simulink model "Experiment_AERO_pitch_channel"  (Simulink 9.1)
settings: Solver=ode4  StartTime=0.0  StopTime=35  FixedStep=0.001  RelTol=1e-3  EnableMultiTasking=on
InitFcn:
  | Parameters_and_initial_conditions
values from neighbouring files (symbols this model uses):
  a1 = -Ksp/Jp    (= -3.27334590734)    [Parameters_and_initial_conditions.m]
  a2 = -Dp/Jp    (= -0.354944459971)    [Parameters_and_initial_conditions.m]
  alpha1 = 0.5    [Parameters_and_initial_conditions.m]
  alpha2 = 0.25    [Parameters_and_initial_conditions.m]
  beta1 = 1    [Parameters_and_initial_conditions.m]
  beta1_HGOB = 3/eps    (= 300)    [Parameters_and_initial_conditions.m]
  beta2 = 1/(2*stepsize^0.5)    (= 1.58113883008)    [Parameters_and_initial_conditions.m]
  beta2_HGOB = 3/(eps^2)    (= 30000)    [Parameters_and_initial_conditions.m]
  beta3 = 2/(25*stepsize^1.2)    (= 1.26791455397)    [Parameters_and_initial_conditions.m]
  beta3_HGOB = 1/(eps^3)    (= 1000000)    [Parameters_and_initial_conditions.m]
  delta = 10    [Parameters_and_initial_conditions.m]
  Dp = 0.007768621416960    (= 0.00776862141696)    [Parameters_and_initial_conditions.m]
  Dp_static = Dp*0.05    (= 0.000388431070848)    [Parameters_and_initial_conditions.m]
  Dy = 0.0220    (= 0.022)    [Parameters_and_initial_conditions.m]
  Jp = J_body + 2*J_prop    (= 0.0218868648283)    [Parameters_and_initial_conditions.m]
  Jy = J_body + 2*J_prop + J_yoke    (= 0.0219920648283)    [Parameters_and_initial_conditions.m]
  kd = 3    [Parameters_and_initial_conditions.m]
  kp = 5    [Parameters_and_initial_conditions.m]
  Kpp = 9.971955650940002e-04    (= 0.000997195565094)    [Parameters_and_initial_conditions.m]
  Kpy = 0.0021    [Parameters_and_initial_conditions.m]
  Ksp = 0.071643279410402    (= 0.0716432794104)    [Parameters_and_initial_conditions.m]
  Kyp = -0.0027    [Parameters_and_initial_conditions.m]
  Kyy = 0.0022    [Parameters_and_initial_conditions.m]
  PitchAxisEnable = 1    [Parameters_and_initial_conditions.m]
  PitchMotorEnable = 1    [Parameters_and_initial_conditions.m]
  psi_dot_initial = 0.0    (= 0)    [Parameters_and_initial_conditions.m]
  psi_initial = 0.0    (= 0)    [Parameters_and_initial_conditions.m]
  theta_dot_initial = 0.0    (= 0)    [Parameters_and_initial_conditions.m]
  theta_initial = 0.0    (= 0)    [Parameters_and_initial_conditions.m]
  YawAxisEnable = 0    [Parameters_and_initial_conditions.m]
  YawMotorEnable = 0    [Parameters_and_initial_conditions.m]
libraries: quarc_library x9, simulink_extras x5, quanser_aero x1
settings Model: Creator=MLevis  LastModifiedBy=DELL  SimulationMode=external  ExtModeTrigDuration=5000
settings SolverCC: PositivePriorityOrder=on
settings DataIOCC: LimitDataPoints=on
settings DebuggingCC: UnderspecifiedInitializationDetection=Simplified  MergeDetectMultiDrivingBlocksExec=error  SolverPrmCheckMsg=warning
settings RTWCC: SystemTargetFile=quarc_win64.tlc  TemplateMakefile=quarc_default_tmf  Description=QUARC Win64 Target
settings STFCustomTargetCC: TargetPreCompLibLocation=C:\PROGRA~3\QUARC\lib\2018a\win64\release  ConcurrentExecutionCompliant=on  GeneratePreprocessorConditionals=Disable all  SystemTargetFile=quarc_win64.tlc
settings GRTTargetCC: TargetPreCompLibLocation=C:\PROGRA~3\QUARC\lib\2018a\win64\release  ParMdlRefBuildCompliant=off  CompOptLevelCompliant=off  GeneratePreprocessorConditionals=Disable all  MatFileLogging=off  CPPClassGenCompliant=off  UseToolchainInfoCompliant=off  ExtMode=on  ExtModeMexFile=quarc_comm
settings ConfigComp: CovSFcnEnable=off

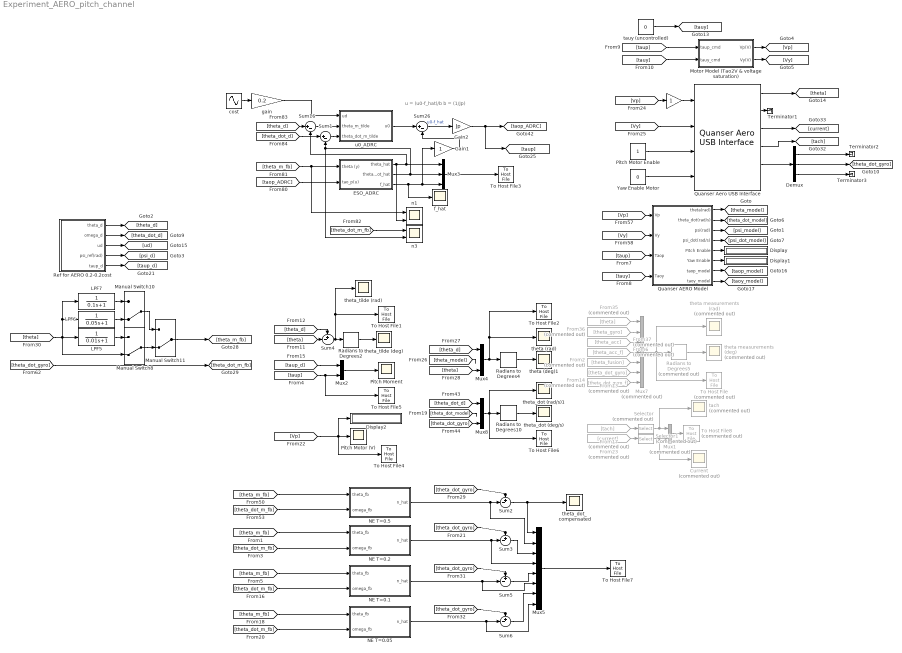
== system Experiment_AERO_pitch_channel ==
  note: u = (u0-f_hat)/b
      | b = (1/Jp)
  " " : Gain
  Current : Scope  Commented=on
  Demux : Demux  Outputs=3
  Display : Display
  Display1 : Display
  Display2 : Display
  ESO_ADRC : Subsystem
  From13 : From  Commented=on  GotoTag=theta_dot_gyro
  From14 : From  Commented=on  GotoTag=theta_dot_gyro_f
  From17 : From  Commented=on  GotoTag=tach
  From2 : From  Commented=on  GotoTag=theta_fusion
  From23 : From  Commented=on  GotoTag=current
  From35 : From  Commented=on  GotoTag=theta
  From36 : From  Commented=on  GotoTag=theta_gyro
  From37 : From  Commented=on  GotoTag=theta_acc
  From6 : From  Commented=on  GotoTag=theta_acc_f
  Gain1 : Gain
  Gain2 : Gain  Gain=Jp
  LPF5 : TransferFcn  Denominator=[0.01 1]
  LPF6 : TransferFcn  Denominator=[0.05 1]
  LPF7 : TransferFcn  Denominator=[0.1 1]
  Manual Switch10 : ManualSwitch  CurrentSetting=0
  Manual Switch11 : ManualSwitch  CurrentSetting=0
  Manual Switch8 : ManualSwitch  CurrentSetting=0
  Motor Model (Tao2V & voltage saturation) : Subsystem
  Mux1 : Mux  Commented=on  Inputs=2
  Mux2 : Mux  Inputs=2
  Mux3 : Mux  Inputs=3
  Mux4 : Mux  Inputs=3
  Mux5 : Mux  Inputs=8
  Mux7 : Mux  Commented=on  Inputs=7
  Mux8 : Mux  Inputs=3
  NE T=0.05 : Subsystem
  NE T=0.1 : Subsystem
  NE T=0.2 : Subsystem
  NE T=0.5 : Subsystem
  Pitch Moment : Scope
  Pitch Motor (V) : Scope
  Pitch Motor Enable : Constant
  Quanser AERO Model : Subsystem
  Quanser Aero USB Interface : quanser_aero/Quanser Aero USB Interface
  Radians to Degrees10 : simulink_extras/Transformations/Radians to Degrees
  Radians to Degrees2 : simulink_extras/Transformations/Radians to Degrees
  Radians to Degrees4 : simulink_extras/Transformations/Radians to Degrees
  Radians to Degrees5 : simulink_extras/Transformations/Radians to Degrees  Commented=on
  Ref for AERO 0.2-0.2cost : Subsystem
  Selector : Selector  Commented=on  InputPortWidth=2  IndexOptions=Index vector (dialog)  Indices=[1]  OutputSizes=1
  Selector1 : Selector  Commented=on  InputPortWidth=2  IndexOptions=Index vector (dialog)  Indices=[1]  OutputSizes=1
  Sum1 : Sum  Inputs=|+-
  Sum16 : Sum  Inputs=|+-
  Sum{2..6} (5 alike) : Sum  Inputs=+-|
  Sum26 : Sum  Inputs=|+-
  Terminator1 : Terminator
  Terminator2 : Terminator
  Terminator3 : Terminator
  To Host File : quarc_library/Sinks/To Host/To Host File  Commented=on  file_name=Log_Sensor_Measurements.mat  variable_name=Log_Sensor_Measurements  decimation=1  sample_time=-1  file_format=MAT-file v.5  options=No header or footer  append=off  final_file_name=Log_Sensor_Measurements.mat  bitrate=2000000
  To Host File1 : quarc_library/Sinks/To Host/To Host File  file_name=Log_Tracking_Err.mat  variable_name=Log_Tracking_Err  decimation=1  sample_time=-1  file_format=MAT-file v.5  options=No header or footer  append=off  final_file_name=Log_Tracking_Err.mat  bitrate=2000000
  To Host File2 : quarc_library/Sinks/To Host/To Host File  file_name=Log_Theta_Response.mat  variable_name=Log_Theta_Response  decimation=1  sample_time=-1  file_format=MAT-file v.5  options=No header or footer  append=off  final_file_name=Log_Theta_Response.mat  bitrate=2000000
  To Host File3 : quarc_library/Sinks/To Host/To Host File  file_name=Log_ESO.mat  variable_name=Log_ESO  decimation=1  sample_time=-1  file_format=MAT-file v.5  options=No header or footer  append=off  final_file_name=Log_ESO.mat  bitrate=2000000
  To Host File4 : quarc_library/Sinks/To Host/To Host File  file_name=Log_Input_Voltage.mat  variable_name=Log_Input_Voltage  decimation=1  sample_time=-1  file_format=MAT-file v.5  options=No header or footer  append=off  final_file_name=Log_Input_Voltage.mat  bitrate=2000000
  To Host File5 : quarc_library/Sinks/To Host/To Host File  file_name=Log_Input_Torque.mat  variable_name=Log_Input_Torque  decimation=1  sample_time=-1  file_format=MAT-file v.5  options=No header or footer  append=off  final_file_name=Log_Input_Torque.mat  bitrate=2000000
  To Host File6 : quarc_library/Sinks/To Host/To Host File  file_name=Log_Theta_dot_Response.mat  variable_name=Log_Theta_dot_Response  decimation=1  sample_time=-1  file_format=MAT-file v.5  options=No header or footer  append=off  final_file_name=Log_Theta_dot_Response.mat  bitrate=2000000
  To Host File7 : quarc_library/Sinks/To Host/To Host File  file_name=Log_Theta_dot_NE_estimation.mat  variable_name=Log_Theta_dot_NE_estimation  decimation=1  sample_time=-1  file_format=MAT-file v.5  options=No header or footer  append=off  final_file_name=Log_Theta_dot_NE_estimation.mat  bitrate=2000000
  To Host File8 : quarc_library/Sinks/To Host/To Host File  Commented=on  file_name=Log_Tach_Current.mat  variable_name=Log_Tach_Current  decimation=1  sample_time=-1  file_format=MAT-file v.5  options=No header or footer  append=off  final_file_name=Log_Tach_Current.mat  bitrate=2000000
  Yaw Enable Motor : Constant  Value=0
  cost : Sin  Phase=pi/2  SampleTime=0
  f_hat : Scope
  gain : Gain  Gain=0.2
  n1 : Scope  NumInputPorts=2
  n3 : Scope  NumInputPorts=2
  tach : Scope  Commented=on
  tauy (uncontrolled) : Constant  Value=0
  theta (deg)1 : Scope
  theta (rad) : Scope
  theta measurements (deg) : Scope  Commented=on
  theta measurements (rad) : Scope  Commented=on
  theta_dot (deg/s) : Scope
  theta_dot (rad/s)1 : Scope
  theta_dot_compensated : Scope
  theta_tilde (deg) : Scope
  theta_tilde (rad) : Scope
  u0_ADRC : Subsystem
  wires:
  Quanser AERO Model/3(psi(rad)) -> [psi_model]
  Quanser AERO Model/1(theta(rad)) -> [theta_model]
  Mux2/1 -> Pitch Moment/1
  Quanser AERO Model/2(theta_dot(rad/s)) -> [theta_dot_model]
  Quanser AERO Model/4(psi_dot(rad/s)) -> [psi_dot_model]
  Quanser AERO Model/5(Pitch Enable) -> Display/1
  Quanser AERO Model/6(Yaw Enable) -> Display1/1
  Motor Model (Tao2V & voltage saturation)/1(Vp(V)) -> [Vp]
  Motor Model (Tao2V & voltage saturation)/2(Vy(V)) -> [Vy]
  [tauy] -> Motor Model (Tao2V & voltage saturation)/2(tauy_cmd)
  [taup] -> Motor Model (Tao2V & voltage saturation)/1(taup_cmd)
  [theta_d] -> Sum4/1
  [theta] -> Sum4/2
  Sum4/1 -> To Host File1/1, theta_tilde (rad)/1, Radians to Degrees2/1
  Radians to Degrees2/1 -> theta_tilde (deg)/1
  [taup] -> To Host File5/1, Mux2/2
  [taup_d] -> Mux2/1
  tauy (uncontrolled)/1 -> [tauy]
  [Vp] -> Display2/1, To Host File4/1, Pitch Motor (V)/1
  Quanser Aero USB Interface/5 -> Demux/1
  Yaw Enable Motor/1 -> Quanser Aero USB Interface/4
  Quanser Aero USB Interface/4 -> [tach]
  Quanser Aero USB Interface/1 -> [theta]
  Demux/3 -> Terminator3/1
  Pitch Motor Enable/1 -> Quanser Aero USB Interface/3
  Quanser Aero USB Interface/3 -> [current]
  [Vy] -> Quanser Aero USB Interface/2
  Demux/1 -> Terminator2/1
  Demux/2 -> [theta_dot_gyro]
  Quanser Aero USB Interface/2 -> Terminator1/1
  " "/1 -> Quanser Aero USB Interface/1
  Radians to Degrees4/1 -> theta (deg)1/1
  [theta_model] -> ?
  [theta_d] -> Mux4/1
  [theta] -> Mux4/3
  Quanser AERO Model/7(taop_model) -> [taop_model]
  Quanser AERO Model/8(taoy_model) -> [taoy_model]
  From35/1 -> Mux7/1
  From36/1 -> Mux7/2
  From37/1 -> Mux7/3
  Radians to Degrees5/1 -> theta measurements (deg)/1
  Radians to Degrees10/1 -> theta_dot (deg/s)/1
  [theta_dot_model] -> ?
  Mux8/1 -> Radians to Degrees10/1, To Host File6/1, theta_dot (rad/s)1/1
  [theta_dot_gyro] -> Mux8/3
  [theta_dot_d] -> Mux8/1
  From6/1 -> Mux7/4
  Mux7/1 -> To Host File/1, theta measurements (rad)/1, Radians to Degrees5/1
  [taup] -> Quanser AERO Model/3(Taop)
  [tauy] -> Quanser AERO Model/4(Taoy)
  [Vp] -> Quanser AERO Model/1(Vp)
  [Vy] -> Quanser AERO Model/2(Vy)
  [theta_dot_gyro] -> [theta_dot_m_fb]
  Mux4/1 -> Radians to Degrees4/1, To Host File2/1, theta (rad)/1
  From2/1 -> Mux7/5
  From13/1 -> Mux7/6
  From14/1 -> Mux7/7
  From17/1 -> Selector/1
  Mux1/1 -> To Host File8/1
  From23/1 -> Selector1/1
  Selector/1 -> tach/1, Mux1/1
  Selector1/1 -> Current/1, Mux1/2
  Ref for AERO 0.2-0.2cost/1(theta_d) -> [theta_d]
  Ref for AERO 0.2-0.2cost/2(omega_d) -> [theta_dot_d]
  Ref for AERO 0.2-0.2cost/4(psi_ref(rad)) -> [psi_d]
  Ref for AERO 0.2-0.2cost/3(ud) -> [ud]
  Manual Switch11/1 -> [theta_m_fb]
  [theta] -> LPF5/1, Manual Switch8/2, LPF7/1, LPF6/1
  Ref for AERO 0.2-0.2cost/5(taup_d) -> [taup_d]
  LPF5/1 -> Manual Switch8/1
  LPF6/1 -> Manual Switch10/2
  LPF7/1 -> Manual Switch10/1
  Manual Switch10/1 -> Manual Switch11/1
  Manual Switch8/1 -> Manual Switch11/2
  [Vp] -> " "/1
  ESO_ADRC/3(f_hat) -> f_hat/1, Gain1/1, Mux3/3
  ESO_ADRC/1(theta_hat) -> n1/2, Sum16/2, Mux3/1
  [theta_dot_m_fb] -> n3/1
  u0_ADRC/1(u0) -> Sum26/1
  Gain1/1 -> Sum26/2
  Sum26/1 -> Gain2/1  "u0-f_hat"
  [taop_ADRC] -> ESO_ADRC/2(tao_p(u))
  [theta_d] -> Sum16/1
  ESO_ADRC/2(theta_dot_hat) -> Mux3/2, n3/2, Sum1/2
  Gain2/1 -> [taup], [taop_ADRC]
  [theta_m_fb] -> n1/1, ESO_ADRC/1(theta (y))
  [theta_dot_d] -> Sum1/1
  Sum16/1 -> u0_ADRC/2(theta_m_tilde)
  Sum1/1 -> u0_ADRC/3(theta_dot_m_tilde)
  Mux3/1 -> To Host File3/1
  cost/1 -> gain/1
  gain/1 -> u0_ADRC/1(ud)
  [theta_m_fb] -> NE T=0.5/1(theta_fb)
  [theta_dot_m_fb] -> NE T=0.5/2(omega_fb)
  Sum2/1 -> Mux5/1, theta_dot_compensated/1
  [theta_dot_gyro] -> Sum2/1
  Mux5/1 -> To Host File7/1
  NE T=0.5/1(n_hat) -> Mux5/2, Sum2/2
  [theta_dot_m_fb] -> NE T=0.2/2(omega_fb)
  [theta_m_fb] -> NE T=0.2/1(theta_fb)
  [theta_dot_m_fb] -> NE T=0.1/2(omega_fb)
  [theta_m_fb] -> NE T=0.1/1(theta_fb)
  [theta_dot_m_fb] -> NE T=0.05/2(omega_fb)
  [theta_m_fb] -> NE T=0.05/1(theta_fb)
  [theta_dot_gyro] -> Sum3/1
  [theta_dot_gyro] -> Sum5/1
  NE T=0.2/1(n_hat) -> Mux5/4, Sum3/2
  NE T=0.05/1(n_hat) -> Mux5/8, Sum6/2
  [theta_dot_gyro] -> Sum6/1
  NE T=0.1/1(n_hat) -> Mux5/6, Sum5/2
  Sum3/1 -> Mux5/3
  Sum5/1 -> Mux5/5
  Sum6/1 -> Mux5/7

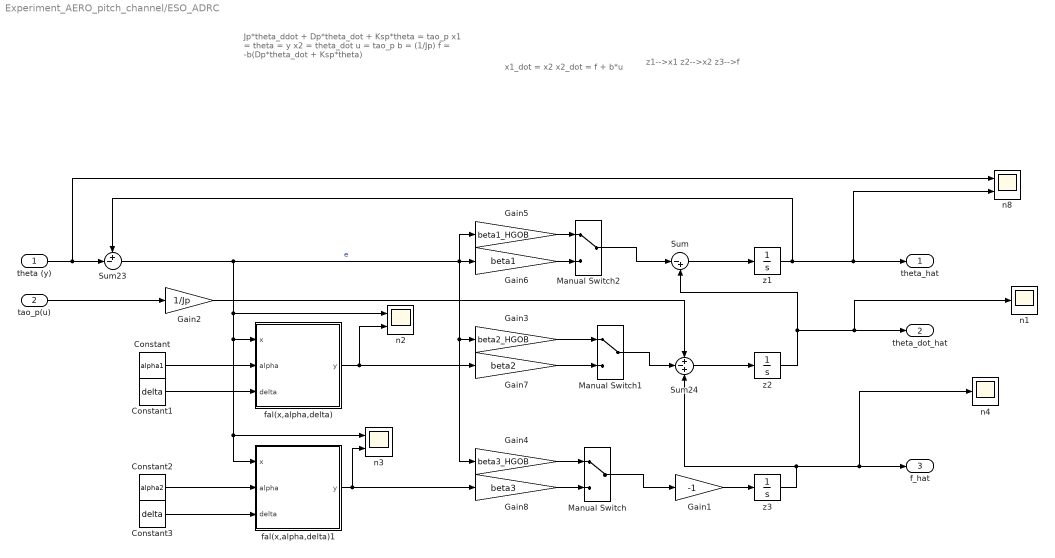
== system Experiment_AERO_pitch_channel/ESO_ADRC ==
  note: z1-->x1
      | z2-->x2
      | z3-->f
  note: x1_dot = x2
      | x2_dot = f + b*u
  note: Jp*theta_ddot + Dp*theta_dot + Ksp*theta = tao_p
      | x1 = theta = y
      | x2 = theta_dot
      | u = tao_p
      | b = (1/Jp)
      | f = -b(Dp*theta_dot + Ksp*theta)
  theta (y) : Inport
  tao_p(u) : Inport  Port=2
  Constant : Constant  Value=alpha1
  Constant1 : Constant  Value=delta
  Constant2 : Constant  Value=alpha2
  Constant3 : Constant  Value=delta
  Gain1 : Gain  Gain=-1
  Gain2 : Gain  Gain=1/Jp
  Gain3 : Gain  Gain=beta2_HGOB
  Gain4 : Gain  Gain=beta3_HGOB
  Gain5 : Gain  Gain=beta1_HGOB
  Gain6 : Gain  Gain=beta1
  Gain7 : Gain  Gain=beta2
  Gain8 : Gain  Gain=beta3
  Manual Switch : ManualSwitch
  Manual Switch1 : ManualSwitch
  Manual Switch2 : ManualSwitch
  Sum : Sum  Inputs=|-+
  Sum23 : Sum  Inputs=+-|
  Sum24 : Sum  Inputs=+-+
  fal(x,alpha,delta) : MATLAB Function  TreatAsAtomicUnit=on
  fal(x,alpha,delta)1 : MATLAB Function  TreatAsAtomicUnit=on
  n1 : Scope
  n2 : Scope  NumInputPorts=2
  n3 : Scope  NumInputPorts=2
  n4 : Scope
  n8 : Scope  NumInputPorts=2
  z1 : Integrator
  z2 : Integrator
  z3 : Integrator
  theta_hat : Outport
  theta_dot_hat : Outport  Port=2
  f_hat : Outport  Port=3
  wires:
  z2/1 -> Sum/2, n1/1, theta_dot_hat/1
  Sum23/1 -> Gain6/1, Gain5/1, Gain3/1, Gain4/1, n2/1, n3/1, fal(x,alpha,delta)1/1(x), fal(x,alpha,delta)/1(x)  "e"
  Gain7/1 -> Manual Switch1/2
  Gain6/1 -> Manual Switch2/2
  z3/1 -> Sum24/3, n4/1, f_hat/1
  Sum24/1 -> z2/1
  Sum/1 -> z1/1
  z1/1 -> n8/2, theta_hat/1, Sum23/1
  Gain8/1 -> Manual Switch/2
  theta (y)/1 -> n8/1, Sum23/2
  tao_p(u)/1 -> Gain2/1
  Gain1/1 -> z3/1
  Gain2/1 -> Sum24/1
  fal(x,alpha,delta)/1(y) -> Gain7/1, n2/2
  Constant/1 -> fal(x,alpha,delta)/2(alpha)
  Constant1/1 -> fal(x,alpha,delta)/3(delta)
  Constant3/1 -> fal(x,alpha,delta)1/3(delta)
  Constant2/1 -> fal(x,alpha,delta)1/2(alpha)
  fal(x,alpha,delta)1/1(y) -> Gain8/1, n3/2
  Gain4/1 -> Manual Switch/1
  Manual Switch/1 -> Gain1/1
  Gain3/1 -> Manual Switch1/1
  Manual Switch1/1 -> Sum24/2
  Gain5/1 -> Manual Switch2/1
  Manual Switch2/1 -> Sum/1

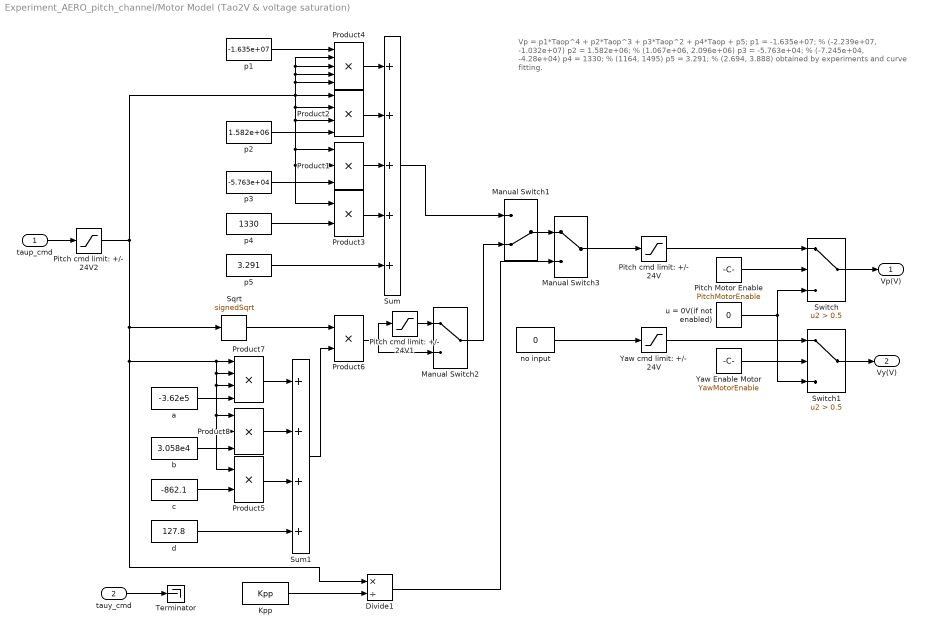
== system Experiment_AERO_pitch_channel/Motor Model (Tao2V & voltage saturation) ==
  note: Vp = p1*Taop^4 + p2*Taop^3 + p3*Taop^2 + p4*Taop + p5;
      | p1 = -1.635e+07; % (-2.239e+07, -1.032e+07)
      | p2 = 1.582e+06; % (1.067e+06, 2.096e+06)
      | p3 = -5.763e+04; % (-7.245e+04, -4.28e+04)
      | p4 = 1330; % (1164, 1495)
      | p5 = 3.291; % (2.694, 3.888)
      |
      | obtained by experiments and curve fitting.
  taup_cmd : Inport
  tauy_cmd : Inport  Port=2
  Divide1 : Product  Inputs=*/
  Kpp : Constant  Value=Kpp
  Manual Switch1 : ManualSwitch  CurrentSetting=0
  Manual Switch2 : ManualSwitch
  Manual Switch3 : ManualSwitch
  Pitch Motor Enable : Constant  Value=PitchMotorEnable
  Pitch cmd limit: +/- 24V : Saturate  UpperLimit=24  LowerLimit=-24
  Pitch cmd limit: +/- 24V1 : Saturate  UpperLimit=24  LowerLimit=0
  Pitch cmd limit: +/- 24V2 : Saturate  UpperLimit=0.05  LowerLimit=0
  Product1 : Product  Inputs=3
  Product2 : Product  Inputs=4
  Product3 : Product
  Product4 : Product  Inputs=5
  Product5 : Product
  Product6 : Product
  Product7 : Product  Inputs=4
  Product8 : Product  Inputs=3
  Sqrt : Sqrt  Operator=signedSqrt  SaturateOnIntegerOverflow=on
  Sum : Sum  Inputs=+++++
  Sum1 : Sum  Inputs=++++
  Switch : Switch  Criteria=u2 > Threshold  Threshold=0.5
  Switch1 : Switch  Criteria=u2 > Threshold  Threshold=0.5
  Terminator : Terminator
  Yaw Enable Motor : Constant  Value=YawMotorEnable
  Yaw cmd limit: +/- 24V : Saturate  UpperLimit=24  LowerLimit=-24
  a : Constant  Value=-3.62e5
  b : Constant  Value=3.058e4
  c : Constant  Value=-862.1
  d : Constant  Value=127.8
  no input : Constant  Value=0
  p1 : Constant  Value=-1.635e+07
  p2 : Constant  Value=1.582e+06
  p3 : Constant  Value=-5.763e+04
  p4 : Constant  Value=1330
  p5 : Constant  Value=3.291
  u = 0V(if not enabled) : Constant  Value=0
  Vp(V) : Outport
  Vy(V) : Outport  Port=2
  wires:
  Pitch Motor Enable/1 -> Switch/2
  Yaw Enable Motor/1 -> Switch1/2
  Switch/1 -> Vp(V)/1
  Switch1/1 -> Vy(V)/1
  Yaw cmd limit: +/- 24V/1 -> Switch1/1
  Pitch cmd limit: +/- 24V/1 -> Switch/1
  u = 0V(if not enabled)/1 -> Switch1/3, Switch/3
  tauy_cmd/1 -> Terminator/1
  p2/1 -> Product2/4
  no input/1 -> Yaw cmd limit: +/- 24V/1
  Product2/1 -> Sum/2
  p3/1 -> Product1/3
  p4/1 -> Product3/2
  Kpp/1 -> Divide1/2
  Product1/1 -> Sum/3
  Product3/1 -> Sum/4
  p5/1 -> Sum/5
  Sum/1 -> Manual Switch1/1
  Product4/1 -> Sum/1
  p1/1 -> Product4/1
  Manual Switch3/1 -> Pitch cmd limit: +/- 24V/1
  a/1 -> Product7/4
  b/1 -> Product8/3
  Sum1/1 -> Product6/2
  Sqrt/1 -> Product6/1
  Product6/1 -> Pitch cmd limit: +/- 24V1/1, Manual Switch2/2
  Manual Switch1/1 -> Manual Switch3/1
  Divide1/1 -> Manual Switch3/2
  d/1 -> Sum1/4
  Product7/1 -> Sum1/1
  Product8/1 -> Sum1/2
  Product5/1 -> Sum1/3
  c/1 -> Product5/2
  taup_cmd/1 -> Pitch cmd limit: +/- 24V2/1
  Pitch cmd limit: +/- 24V1/1 -> Manual Switch2/1
  Manual Switch2/1 -> Manual Switch1/2
  Pitch cmd limit: +/- 24V2/1 -> Sqrt/1, Divide1/1, Product7/1, Product7/2, Product7/3, Product8/1, Product8/2, Product5/1, Product4/5, Product4/4, Product4/3, Product4/2, Product2/1, Product3/1, Product1/2, Product1/1, Product2/3, Product2/2

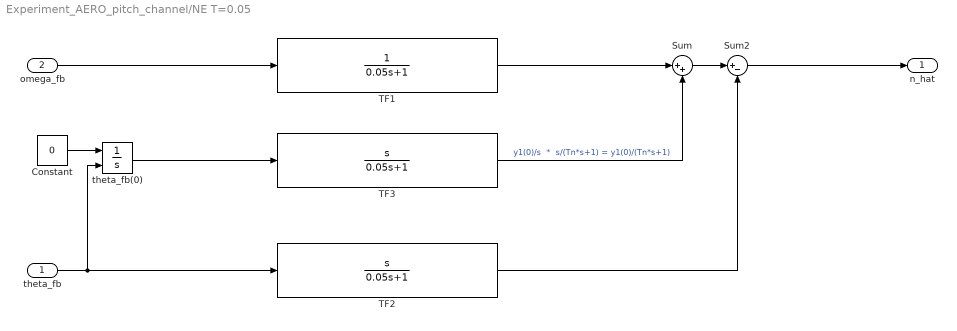
== system Experiment_AERO_pitch_channel/NE T=0.05 ==
  theta_fb : Inport
  omega_fb : Inport  Port=2
  Constant : Constant  Value=0
  Sum : Sum  Inputs=|++
  Sum2 : Sum  Inputs=|+-
  TF1 : TransferFcn  Denominator=[0.05 1]
  TF2 : TransferFcn  Numerator=[1 0]  Denominator=[0.05 1]
  TF3 : TransferFcn  Numerator=[1 0]  Denominator=[0.05 1]
  theta_fb(0) : Integrator  InitialConditionSource=external
  n_hat : Outport
  wires:
  TF3/1 -> Sum/2  "y1(0)/s  *  s/(Tn*s+1) = y1(0)/(Tn*s+1)"
  Sum/1 -> Sum2/1
  omega_fb/1 -> TF1/1
  theta_fb(0)/1 -> TF3/1
  Constant/1 -> theta_fb(0)/1
  TF1/1 -> Sum/1
  TF2/1 -> Sum2/2
  Sum2/1 -> n_hat/1
  theta_fb/1 -> theta_fb(0)/2, TF2/1

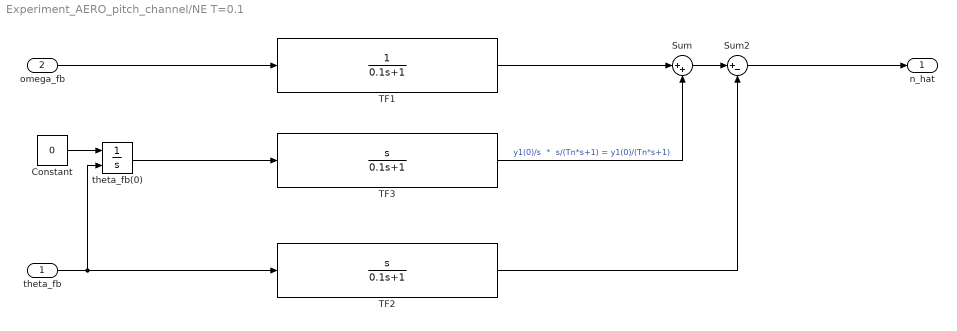
== system Experiment_AERO_pitch_channel/NE T=0.1 ==
  theta_fb : Inport
  omega_fb : Inport  Port=2
  Constant : Constant  Value=0
  Sum : Sum  Inputs=|++
  Sum2 : Sum  Inputs=|+-
  TF1 : TransferFcn  Denominator=[0.1 1]
  TF2 : TransferFcn  Numerator=[1 0]  Denominator=[0.1 1]
  TF3 : TransferFcn  Numerator=[1 0]  Denominator=[0.1 1]
  theta_fb(0) : Integrator  InitialConditionSource=external
  n_hat : Outport
  wires:
  theta_fb/1 -> TF2/1, theta_fb(0)/2
  Sum2/1 -> n_hat/1
  TF2/1 -> Sum2/2
  TF1/1 -> Sum/1
  Constant/1 -> theta_fb(0)/1
  theta_fb(0)/1 -> TF3/1
  omega_fb/1 -> TF1/1
  Sum/1 -> Sum2/1
  TF3/1 -> Sum/2  "y1(0)/s  *  s/(Tn*s+1) = y1(0)/(Tn*s+1)"

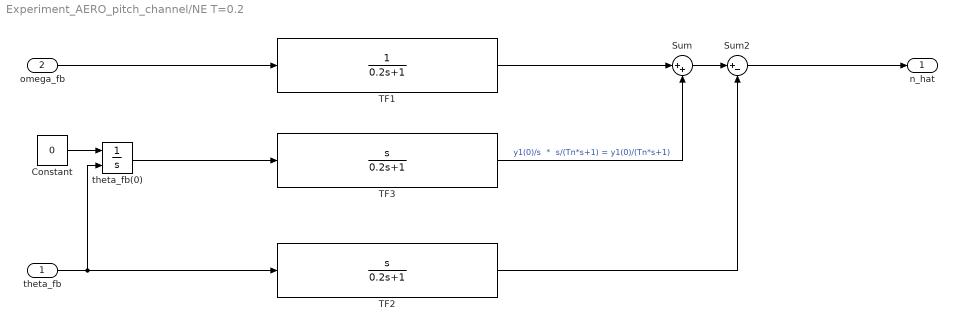
== system Experiment_AERO_pitch_channel/NE T=0.2 ==
  theta_fb : Inport
  omega_fb : Inport  Port=2
  Constant : Constant  Value=0
  Sum : Sum  Inputs=|++
  Sum2 : Sum  Inputs=|+-
  TF1 : TransferFcn  Denominator=[0.2 1]
  TF2 : TransferFcn  Numerator=[1 0]  Denominator=[0.2 1]
  TF3 : TransferFcn  Numerator=[1 0]  Denominator=[0.2 1]
  theta_fb(0) : Integrator  InitialConditionSource=external
  n_hat : Outport
  wires:
  TF3/1 -> Sum/2  "y1(0)/s  *  s/(Tn*s+1) = y1(0)/(Tn*s+1)"
  Sum/1 -> Sum2/1
  omega_fb/1 -> TF1/1
  theta_fb(0)/1 -> TF3/1
  Constant/1 -> theta_fb(0)/1
  TF1/1 -> Sum/1
  TF2/1 -> Sum2/2
  Sum2/1 -> n_hat/1
  theta_fb/1 -> theta_fb(0)/2, TF2/1

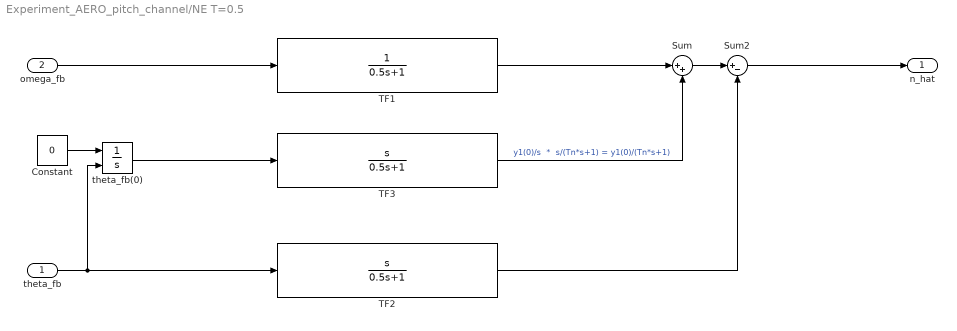
== system Experiment_AERO_pitch_channel/NE T=0.5 ==
  theta_fb : Inport
  omega_fb : Inport  Port=2
  Constant : Constant  Value=0
  Sum : Sum  Inputs=|++
  Sum2 : Sum  Inputs=|+-
  TF1 : TransferFcn  Denominator=[0.5 1]
  TF2 : TransferFcn  Numerator=[1 0]  Denominator=[0.5 1]
  TF3 : TransferFcn  Numerator=[1 0]  Denominator=[0.5 1]
  theta_fb(0) : Integrator  InitialConditionSource=external
  n_hat : Outport
  wires:
  theta_fb/1 -> TF2/1, theta_fb(0)/2
  Sum2/1 -> n_hat/1
  TF2/1 -> Sum2/2
  TF1/1 -> Sum/1
  Constant/1 -> theta_fb(0)/1
  theta_fb(0)/1 -> TF3/1
  omega_fb/1 -> TF1/1
  Sum/1 -> Sum2/1
  TF3/1 -> Sum/2  "y1(0)/s  *  s/(Tn*s+1) = y1(0)/(Tn*s+1)"

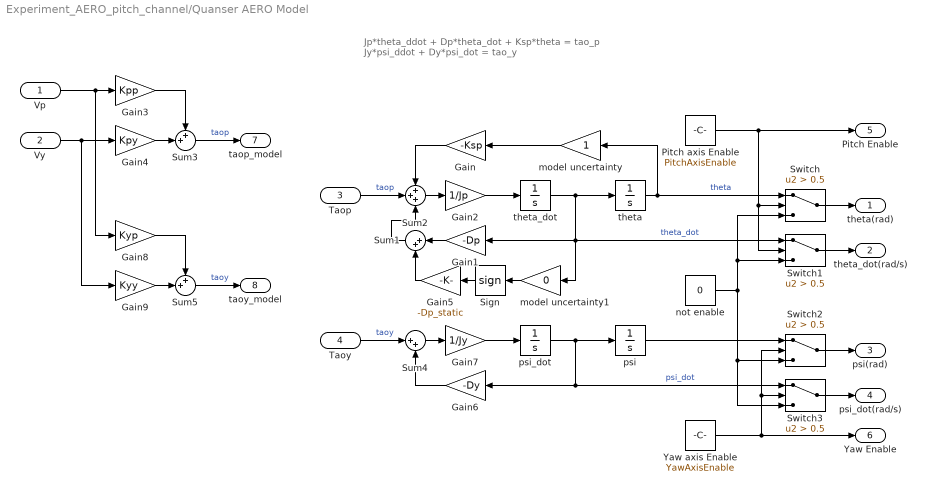
== system Experiment_AERO_pitch_channel/Quanser AERO Model ==
  note: Jp*theta_ddot + Dp*theta_dot + Ksp*theta = tao_p
      | Jy*psi_ddot + Dy*psi_dot = tao_y
  Vp : Inport
  Vy : Inport  Port=2
  Taop : Inport  Port=3
  Taoy : Inport  Port=4
  Gain : Gain  Gain=-Ksp
  Gain1 : Gain  Gain=-Dp
  Gain2 : Gain  Gain=1/Jp
  Gain3 : Gain  Gain=Kpp
  Gain4 : Gain  Gain=Kpy
  Gain5 : Gain  Gain=-Dp_static
  Gain6 : Gain  Gain=-Dy
  Gain7 : Gain  Gain=1/Jy
  Gain8 : Gain  Gain=Kyp
  Gain9 : Gain  Gain=Kyy
  Pitch axis Enable : Constant  Value=PitchAxisEnable
  Sign : Signum
  Sum1 : Sum  Inputs=|++
  Sum2 : Sum  Inputs=+++
  Sum3 : Sum  Inputs=++|
  Sum4 : Sum  Inputs=|++
  Sum5 : Sum  Inputs=++|
  Switch{,1..3} (4 alike) : Switch  Criteria=u2 > Threshold  Threshold=0.5
  Yaw axis Enable : Constant  Value=YawAxisEnable
  model uncertainty : Gain
  model uncertainty1 : Gain  Gain=0
  not enable : Constant  Value=0
  psi : Integrator  InitialCondition=psi_initial
  psi_dot : Integrator  InitialCondition=psi_dot_initial
  theta : Integrator  InitialCondition=theta_initial
  theta_dot : Integrator  InitialCondition=theta_dot_initial
  theta(rad) : Outport
  theta_dot(rad/s) : Outport  Port=2
  psi(rad) : Outport  Port=3
  psi_dot(rad/s) : Outport  Port=4
  Pitch Enable : Outport  Port=5
  Yaw Enable : Outport  Port=6
  taop_model : Outport  Port=7
  taoy_model : Outport  Port=8
  wires:
  theta_dot/1 -> model uncertainty1/1, Gain1/1, Switch1/1, theta/1  "theta_dot"
  theta/1 -> Switch/1, model uncertainty/1  "theta"
  Taop/1 -> Sum2/2  "taop"
  Gain/1 -> Sum2/1
  Gain1/1 -> Sum1/1
  Sum2/1 -> Gain2/1
  Gain2/1 -> theta_dot/1
  Gain3/1 -> Sum3/1
  Gain4/1 -> Sum3/2
  psi_dot/1 -> psi/1, Gain6/1, Switch3/1  "psi_dot"
  psi/1 -> Switch2/1
  Taoy/1 -> Sum4/1  "taoy"
  Sum4/1 -> Gain7/1
  Gain7/1 -> psi_dot/1
  Gain8/1 -> Sum5/1
  Gain9/1 -> Sum5/2
  Vp/1 -> Gain8/1, Gain3/1
  Vy/1 -> Gain9/1, Gain4/1
  Gain6/1 -> Sum4/2
  Pitch axis Enable/1 -> Pitch Enable/1, Switch1/2, Switch/2
  Switch/1 -> theta(rad)/1
  Switch1/1 -> theta_dot(rad/s)/1
  not enable/1 -> Switch1/3, Switch/3, Switch3/3, Switch2/3
  Switch2/1 -> psi(rad)/1
  Switch3/1 -> psi_dot(rad/s)/1
  Yaw axis Enable/1 -> Yaw Enable/1, Switch2/2, Switch3/2
  model uncertainty/1 -> Gain/1
  Sum1/1 -> Sum2/3
  Gain5/1 -> Sum1/2
  Sign/1 -> Gain5/1
  model uncertainty1/1 -> Sign/1
  Sum3/1 -> taop_model/1  "taop"
  Sum5/1 -> taoy_model/1  "taoy"

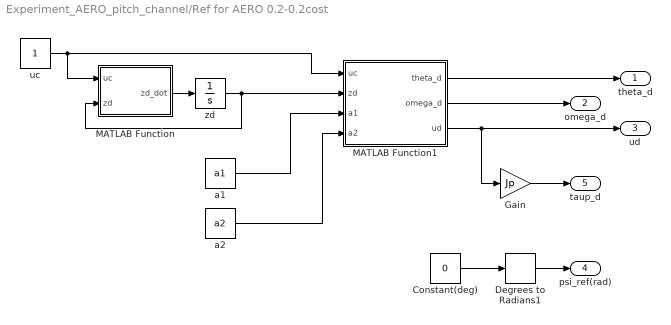
== system Experiment_AERO_pitch_channel/Ref for AERO 0.2-0.2cost ==
  Constant(deg) : Constant  Value=0
  Degrees to Radians1 : simulink_extras/Transformations/Degrees to Radians
  Gain : Gain  Gain=Jp
  MATLAB Function : MATLAB Function  TreatAsAtomicUnit=on
  MATLAB Function1 : MATLAB Function  TreatAsAtomicUnit=on
  a1 : Constant  Value=a1
  a2 : Constant  Value=a2
  uc : Constant
  zd : Integrator  InitialCondition=[0;0]
  theta_d : Outport
  omega_d : Outport  Port=2
  ud : Outport  Port=3
  psi_ref(rad) : Outport  Port=4
  taup_d : Outport  Port=5
  wires:
  MATLAB Function1/1(theta_d) -> theta_d/1
  MATLAB Function1/3(ud) -> ud/1, Gain/1
  MATLAB Function1/2(omega_d) -> omega_d/1
  a2/1 -> MATLAB Function1/4(a2)
  a1/1 -> MATLAB Function1/3(a1)
  uc/1 -> MATLAB Function/1(uc), MATLAB Function1/1(uc)
  zd/1 -> MATLAB Function/2(zd), MATLAB Function1/2(zd)
  MATLAB Function/1(zd_dot) -> zd/1
  Constant(deg)/1 -> Degrees to Radians1/1
  Degrees to Radians1/1 -> psi_ref(rad)/1
  Gain/1 -> taup_d/1

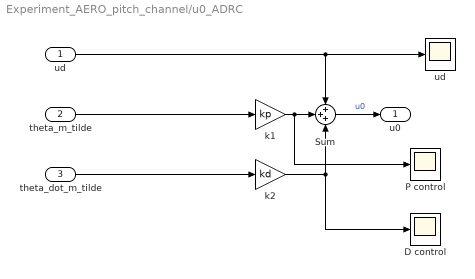
== system Experiment_AERO_pitch_channel/u0_ADRC ==
  ud : Inport
  theta_m_tilde : Inport  Port=2
  theta_dot_m_tilde : Inport  Port=3
  D control : Scope
  P control : Scope
  Sum : Sum  Inputs=+++
  k1 : Gain  Gain=kp
  k2 : Gain  Gain=kd
  "ud " : Scope
  u0 : Outport
  wires:
  ud/1 -> "ud "/1, Sum/1
  theta_m_tilde/1 -> k1/1
  k1/1 -> P control/1, Sum/2
  Sum/1 -> u0/1  "u0"
  theta_dot_m_tilde/1 -> k2/1
  k2/1 -> D control/1, Sum/3

== matlab function Ref for AERO 0.2-0.2cost/MATLAB Function ==
  data: uc input double; zd_dot output double; zd input double
function zd_dot = ref(uc,zd)
Ad = [0 1;-1 0];
Bd = [0; 1];
zd_dot = Ad*zd + Bd*uc;

== matlab function Ref for AERO 0.2-0.2cost/MATLAB Function1 ==
  data: uc input double; zd input double; theta_d output double; omega_d output double; ud output double; a1 input double; a2 input double
function [theta_d, omega_d, ud] = fcn(uc,zd,a1,a2)
Ad = [0 1;-1 0];
Bd = [0; 1];
Cd = [0.2 0];
uc_dot = 0;
w = 0;
theta_d = Cd*zd;
omega_d = Cd*Ad*zd + Cd*Bd*uc;
ud = Cd*Ad*Ad*zd + Cd*Ad*Bd*uc + Cd*Bd*uc_dot - a1*Cd*zd - a2*Cd*Ad*zd - w;

== matlab function ESO_ADRC/fal(x,alpha,delta) ==
  data: x input double; y output double; alpha input double; delta input double
function y = fal(x,alpha,delta)

if (abs(x)<= delta)
   y = x/(delta^(1-alpha));    
else
    y = sign(x)* (abs(x))^alpha;    
end

end

== matlab function ESO_ADRC/fal(x,alpha,delta)1 ==
  data: x input double; y output double; alpha input double; delta input double
function y = fal(x,alpha,delta)

if (abs(x)<= delta)
   y = x/(delta^(1-alpha));    
else
    y = sign(x)* (abs(x))^alpha;    
end

end
